simulink model "Tire_Lateral_Force_Estimation"  (R2022b)
settings: Solver=ode1  StartTime=0.0  StopTime=t_l  FixedStep=0.01  RelTol=1e-3  EnableMultiTasking=on
PostLoadFcn:
  | , if any(exist('dsrtsu_mdlpostloadfcn', 'file') == [2, 3, 6]), try dsrtsu_mdlpostloadfcn('Execute', bdroot); catch fprintf('Error in PostLoadFcn (dsrtsu_mdlpostloadfcn) for model "%s":\n %s\n', bdroot, lasterr); end, end,
values from neighbouring files (symbols this model uses):
  J = 3495    [Cornering_Stiffness_Tuning.m]    (also in Lat_Dynamics_Simul_initialize.m; State_Estimator.m)
  L = Lf+Lr    (= 2.64)    [Cornering_Stiffness_Tuning.m]    (also in Lat_Dynamics_Simul_initialize.m; State_Estimator.m)
  Lf = 1.15    [Cornering_Stiffness_Tuning.m]    (also in Lat_Dynamics_Simul_initialize.m; State_Estimator.m)
  Lr = 1.49    [Cornering_Stiffness_Tuning.m]    (also in Lat_Dynamics_Simul_initialize.m; State_Estimator.m)
  M = 1523    [Cornering_Stiffness_Tuning.m]    (also in Lat_Dynamics_Simul_initialize.m; State_Estimator.m)
settings Model: DSRTSU_INTERNAL_RTI_VER=360  DSRTSU_INTERNAL_RTI_TYPE=rti1005  Creator=5614648  LastModifiedBy=LDW
settings SolverCC: AlgebraicLoopSolver=TrustRegion
settings DataIOCC: LimitDataPoints=on  SaveFormat=Array  SignalLoggingSaveFormat=ModelDataLogs  ReturnWorkspaceOutputs=off
settings OptimizationCC: BlockReduction=off  OptimizeBlockIOStorage=off  BufferReuse=off  GlobalBufferReuse=off  ExpressionFolding=off  ExpressionDepthLimit=2147483647  LocalBlockOutputs=off  LifeSpan=inf
settings DebuggingCC: UnderspecifiedInitializationDetection=Classic  MergeDetectMultiDrivingBlocksExec=none  SolverPrmCheckMsg=warning  FcnCallInpInsideContextMsg=warning  UnconnectedInputMsg=warning  UnconnectedOutputMsg=warning  UnconnectedLineMsg=warning  StateNameClashWarn=warning  SFUnexpectedBacktrackingDiag=warning  SFNoUnconditionalDefaultTransitionDiag=warning  SFExecutionAtInitializationDiag=none  SFMachineParentedDataDiag=warning  ArithmeticOperatorsInVariantConditions=warning
settings HardwareCC: ProdBitPerPointer=32  ProdBitPerSizeT=32  ProdBitPerPtrDiffT=32  ProdLargestAtomicFloat=None  ProdIntDivRoundTo=Undefined  ProdEndianess=Unspecified  ProdWordSize=32  ProdHWDeviceType=32-bit Generic  TargetHWDeviceType=Generic->Custom
settings ModelReferenceCC: PropagateSignalLabelsOutOfModel=off
settings SFSimCC: SimUseLocalCustomCode=off  CustomCodeUndefinedFunction=UseInterfaceOnly
settings RTWCC: Description=dSPACE DS1005 Hardware Platform  SystemTargetFile=rti1005.tlc  MakeCommand=make_rti  TemplateMakefile=rti1005.tmf  RTWUseLocalCustomCode=off
settings CodeAppCC: StateflowObjectComments=on
settings STFCustomTargetCC: CPPClassGenCompliant=on  GRTInterface=on  SystemTargetFile=rti1005.tlc
settings GRTTargetCC: TargetLangStandard=C89/C90 (ANSI)  ParMdlRefBuildCompliant=off  CompOptLevelCompliant=off  ConcurrentExecutionCompliant=off  CombineOutputUpdateFcns=off  MatFileLogging=off  GRTInterface=on  UseToolchainInfoCompliant=off  ExtModeMexFile=noextcomm
settings ConfigComp: CovMetricSettings=dw  CovSaveCumulativeToWorkspaceVar=on  CovSaveSingleToWorkspaceVar=on  CovExternalEMLEnable=off

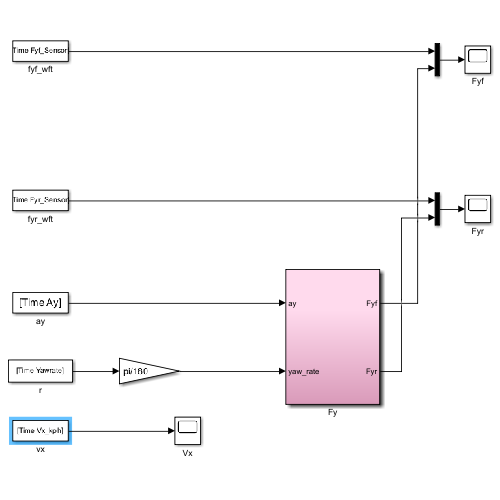
[thumbnail: Simulink's stored preview of the top-level diagram]
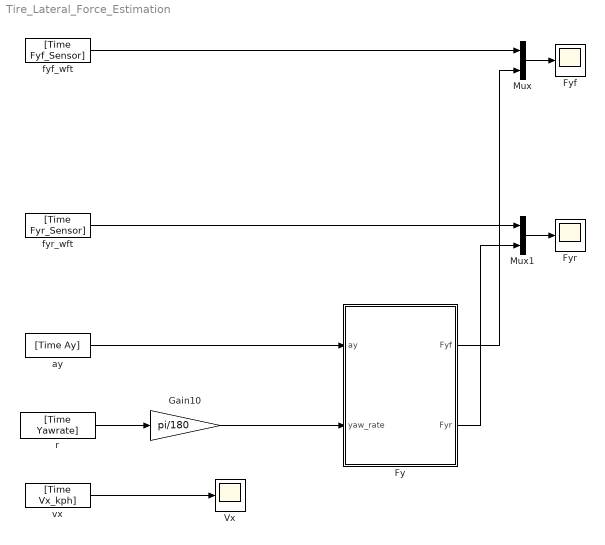
== system Tire_Lateral_Force_Estimation ==
  Fy : Subsystem
  Fyf : Scope
  Fyr : Scope
  Gain10 : Gain  Gain=pi/180
  Mux : Mux  Inputs=2
  Mux1 : Mux  Inputs=2
  Vx : Scope
  ay : FromWorkspace  VariableName=[Time Ay]
  fyf_wft : FromWorkspace  VariableName=[Time Fyf_Sensor]
  fyr_wft : FromWorkspace  VariableName=[Time Fyr_Sensor]
  r : FromWorkspace  VariableName=[Time Yawrate]
  vx : FromWorkspace  VariableName=[Time Vx_kph]
  wires:
  Mux/1 -> Fyf/1
  Mux1/1 -> Fyr/1
  ay/1 -> Fy/1(ay)
  r/1 -> Gain10/1
  Gain10/1 -> Fy/2(yaw_rate)
  Fy/1(Fyf) -> Mux/2
  fyf_wft/1 -> Mux/1
  fyr_wft/1 -> Mux1/1
  Fy/2(Fyr) -> Mux1/2
  vx/1 -> Vx/1

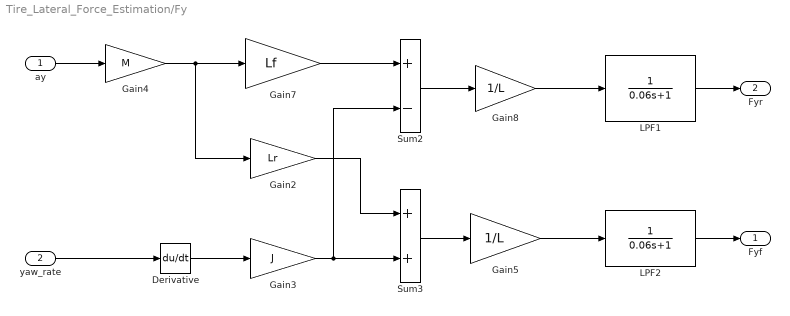
== system Tire_Lateral_Force_Estimation/Fy ==
  ay : Inport
  yaw_rate : Inport  Port=2
  Derivative : Derivative
  Gain2 : Gain  Gain=Lr  SaturateOnIntegerOverflow=on  OutDataTypeStr=Inherit: Same as input  ParamDataTypeStr=Inherit: Same as input
  Gain3 : Gain  Gain=J  SaturateOnIntegerOverflow=on  OutDataTypeStr=Inherit: Same as input  ParamDataTypeStr=Inherit: Same as input
  Gain4 : Gain  Gain=M  SaturateOnIntegerOverflow=on  OutDataTypeStr=Inherit: Same as input  ParamDataTypeStr=Inherit: Same as input
  Gain5 : Gain  Gain=1/L  SaturateOnIntegerOverflow=on  OutDataTypeStr=Inherit: Same as input  ParamDataTypeStr=Inherit: Same as input
  Gain7 : Gain  Gain=Lf  SaturateOnIntegerOverflow=on  OutDataTypeStr=Inherit: Same as input  ParamDataTypeStr=Inherit: Same as input
  Gain8 : Gain  Gain=1/L  SaturateOnIntegerOverflow=on  OutDataTypeStr=Inherit: Same as input  ParamDataTypeStr=Inherit: Same as input
  LPF1 : TransferFcn  Denominator=[0.06 1]
  LPF2 : TransferFcn  Denominator=[0.06 1]
  Sum2 : Sum  Inputs=+-  InputSameDT=on  SaturateOnIntegerOverflow=on  OutDataTypeStr=Inherit: Same as first input
  Sum3 : Sum  InputSameDT=on  SaturateOnIntegerOverflow=on  OutDataTypeStr=Inherit: Same as first input
  Fyf : Outport
  Fyr : Outport  Port=2
  wires:
  ay/1 -> Gain4/1
  Gain4/1 -> Gain2/1, Gain7/1
  Derivative/1 -> Gain3/1
  Gain2/1 -> Sum3/1
  Gain3/1 -> Sum2/2, Sum3/2
  Sum3/1 -> Gain5/1
  Gain7/1 -> Sum2/1
  Sum2/1 -> Gain8/1
  yaw_rate/1 -> Derivative/1
  Gain8/1 -> LPF1/1
  LPF1/1 -> Fyr/1
  Gain5/1 -> LPF2/1
  LPF2/1 -> Fyf/1
